simulink model "Sensor_fusion_4"  (R2024b)
settings: Solver=ode8  StartTime=0.0  StopTime=1000  FixedStep=0.1  RelTol=1e-3
values from neighbouring files (symbols this model uses):
  d = sqrt((Width/2)^2 + (Length/2)^2)    [VariableDeclare.m]
  Delta_t = 0.1    [VariableDeclare.m]
  Length = 0.5    [VariableDeclare.m]
  Wheel_radius = 0.1    [VariableDeclare.m]
  Width = 0.4    [VariableDeclare.m]
undefined symbols (not defined in the file or in its folder): DiscIntNeverNeededParam
libraries: ros2lib x3, simulink x3, sharedTrackingLibrary x1
settings Model: Creator=asrlab  LastModifiedBy=asrlab

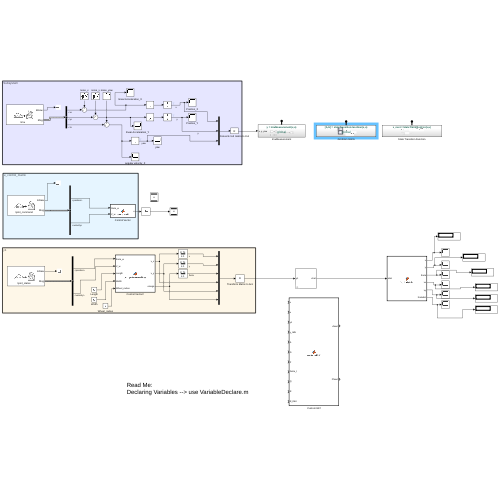
[thumbnail: Simulink's stored preview of the top-level diagram]
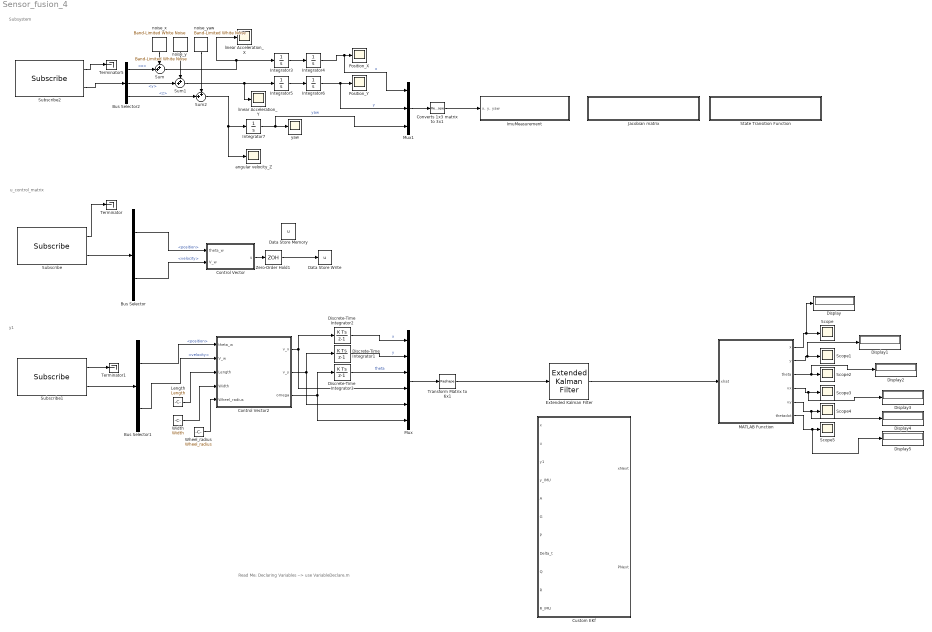
== system Sensor_fusion_4 ==
  note: Read Me:
      | Declaring Variables --> use VariableDeclare.m
  note: y1
  note: u_control_matrix
  note: Subsystem
  Bus Selector : BusSelector  OutputSignals=position,velocity
  Bus Selector1 : BusSelector  OutputSignals=position,velocity
  Bus Selector2 : BusSelector  OutputSignals=linear_acceleration.x,linear_acceleration.y,angular_velocity.z
  Control Vector : MATLAB Function  TreatAsAtomicUnit=on
  Control Vector2 : MATLAB Function  TreatAsAtomicUnit=on
  Converts 1x3 matrix to 3x1 : Reshape  OutputDimensionality=Customize  OutputDimensions=[3,1]
  Custom EKf : MATLAB Function  TreatAsAtomicUnit=on
  Data Store Memory : DataStoreMemory  DataStoreName=u  WriteAfterWriteMsg=warning  ShowAdditionalParam=off  OutDataTypeStr=double  Dimensions=[8 1]
  Data Store Write : DataStoreWrite  DataStoreName=u  IndexOptions=Index vector (dialog)  Indices=1  OutputSizes=1
  Discrete-Time Integrator1 : DiscreteIntegrator  SampleTime=-1  ICPrevOutput=DiscIntNeverNeededParam  ICPrevScaledInput=DiscIntNeverNeededParam
  Discrete-Time Integrator2 : DiscreteIntegrator  SampleTime=-1  ICPrevOutput=DiscIntNeverNeededParam  ICPrevScaledInput=DiscIntNeverNeededParam
  Discrete-Time Integrator3 : DiscreteIntegrator  SampleTime=-1  ICPrevOutput=DiscIntNeverNeededParam  ICPrevScaledInput=DiscIntNeverNeededParam
  Display{,1..5} (6 alike) : Display
  Extended Kalman Filter : sharedTrackingLibrary/Extended Kalman Filter  StateTransitionFcn=StateTransitionFcn  HasStateTransitionJacobianFcn=off  StateTransitionJacobianFcn=stateTransitionJacobian  HasAdditiveProcessNoise=Nonadditive  ProcessNoise=1  HasTimeVaryingProcessNoise=off  HasStateTransitionFcnExtraArgument=0  InitialState=initializationMatrix  InitialStateCovariance=P0  MeasurementFcn1=ImuMeasurement  HasMeasurementJacobianFcn1=off  HasMeasurementEnablePort1=off  HasAdditiveMeasurementNoise1=Nonadditive  MeasurementNoise1=R_IMU  HasTimeVaryingMeasurementNoise1=off  HasMeasurementFcnExtraArgument1=0  HasMeasurementWrapping1=off  MeasurementFcn2=myMeasurementFcn  HasMeasurementJacobianFcn2=off  HasMeasurementEnablePort2=off  HasAdditiveMeasurementNoise2=Additive  MeasurementNoise2=1  HasTimeVaryingMeasurementNoise2=off  HasMeasurementFcnExtraArgument2=0  HasMeasurementWrapping2=off  MeasurementFcn3=myMeasurementFcn  HasMeasurementJacobianFcn3=off  HasMeasurementEnablePort3=off  HasAdditiveMeasurementNoise3=Additive  MeasurementNoise3=1  HasTimeVaryingMeasurementNoise3=off  HasMeasurementFcnExtraArgument3=0  HasMeasurementWrapping3=off  MeasurementFcn4=myMeasurementFcn  HasMeasurementJacobianFcn4=off  HasMeasurementEnablePort4=off  HasAdditiveMeasurementNoise4=Additive  MeasurementNoise4=1  HasTimeVaryingMeasurementNoise4=off  HasMeasurementFcnExtraArgument4=0  HasMeasurementWrapping4=off  MeasurementFcn5=myMeasurementFcn  HasMeasurementJacobianFcn5=off  HasMeasurementEnablePort5=off  HasAdditiveMeasurementNoise5=Additive  MeasurementNoise5=1  HasTimeVaryingMeasurementNoise5=off  HasMeasurementFcnExtraArgument5=0  HasMeasurementWrapping5=off  EnableMultirate=off  StateTransitionFcnSampleTime=1  MeasurementFcn1SampleTime=1  MeasurementFcn2SampleTime=1  MeasurementFcn3SampleTime=1  MeasurementFcn4SampleTime=1  MeasurementFcn5SampleTime=1  UseCurrentEstimator=on  OutputStateCovariance=off  DataType=double  SampleTime=1  NumberOfMeasurements=1
  ImuMeasurement : Subsystem  TreatAsAtomicUnit=on
  Integrator{3..7} (5 alike) : Integrator
  Jacobian matrix : Subsystem  TreatAsAtomicUnit=on
  Length : Constant  Value=Length
  MATLAB Function : MATLAB Function  TreatAsAtomicUnit=on
  Mux : Mux  Inputs=6
  Mux1 : Mux  Inputs=3
  Position_X : Scope
  Position_Y : Scope
  Scope{,1..5} (6 alike) : Scope
  State Transition Function : Subsystem  TreatAsAtomicUnit=on
  Subscribe : ros2lib/Subscribe  topicSource=Select from ROS network  topic=/joint_command  messageType=sensor_msgs/JointState  sampleTime=-1  QOSHistory=Keep last  QOSDepth=1  QOSReliability=Reliable  QOSDurability=Volatile  QOSDeadline=Inf  QOSLifespan=Inf  QOSLiveliness=Automatic  QOSLeaseDuration=Inf  QOSAvoidROSNamespaceConventions=off
  Subscribe1 : ros2lib/Subscribe  topicSource=Select from ROS network  topic=/joint_states  messageType=sensor_msgs/JointState  sampleTime=-1  QOSHistory=Keep last  QOSDepth=1  QOSReliability=Reliable  QOSDurability=Volatile  QOSDeadline=Inf  QOSLifespan=Inf  QOSLiveliness=Automatic  QOSLeaseDuration=Inf  QOSAvoidROSNamespaceConventions=off
  Subscribe2 : ros2lib/Subscribe  topicSource=Select from ROS network  topic=/imu  messageType=sensor_msgs/Imu  sampleTime=-1  QOSHistory=Keep last  QOSDepth=1  QOSReliability=Reliable  QOSDurability=Volatile  QOSDeadline=Inf  QOSLifespan=Inf  QOSLiveliness=Automatic  QOSLeaseDuration=Inf  QOSAvoidROSNamespaceConventions=off
  Sum : Sum  Inputs=++|
  Sum1 : Sum  Inputs=++|
  Sum2 : Sum  Inputs=++|
  Terminator : Terminator
  Terminator1 : Terminator
  Terminator5 : Terminator
  Transform Matrix to 6x1 : Reshape  OutputDimensionality=Customize  OutputDimensions=[6,1]
  Wheel_radius : Constant  Value=Wheel_radius
  Width : Constant  Value=Width
  Zero-Order Hold1 : ZeroOrderHold  SampleTime=Delta_t
  angular velocity_Z : Scope
  linear Acceleration_X : Scope
  linear Acceleration_Y : Scope
  noise_x : simulink/Sources/Band-Limited White Noise  Cov=[0.1]  Ts=0.1  seed=[23341]
  noise_y : simulink/Sources/Band-Limited White Noise  Cov=[0.1]  Ts=0.1  seed=[23341]
  noise_yaw : simulink/Sources/Band-Limited White Noise  Cov=[0.1]  Ts=0.1  seed=[23341]
  yaw : Scope
  wires:
  Zero-Order Hold1/1 -> Data Store Write/1
  Control Vector/1(u) -> Zero-Order Hold1/1
  Bus Selector/1 -> Control Vector/1(theta_w)  "<position>"
  Subscribe/2 -> Bus Selector/1
  Bus Selector/2 -> Control Vector/2(V_w)  "<velocity>"
  Subscribe/1 -> Terminator/1
  Subscribe1/2 -> Bus Selector1/1
  Subscribe1/1 -> Terminator1/1
  Mux/1 -> Transform Matrix to 6x1/1
  Discrete-Time Integrator2/1 -> Mux/1  "x"
  Discrete-Time Integrator1/1 -> Mux/2  "y"
  Discrete-Time Integrator3/1 -> Mux/3  "theta"
  Integrator5/1 -> Integrator6/1
  Bus Selector2/3 -> Sum2/2  "<z>"
  Integrator4/1 -> Mux1/1, Position_X/1  "x"
  Sum2/1 -> Integrator7/1, angular velocity_Z/1
  Mux1/1 -> Converts 1x3 matrix to 3x1/1
  noise_yaw/1 -> Sum2/1
  Subscribe2/1 -> Terminator5/1
  noise_x/1 -> Sum/1
  Sum/1 -> Integrator3/1, linear Acceleration_X/1
  Integrator3/1 -> Integrator4/1
  Subscribe2/2 -> Bus Selector2/1
  noise_y/1 -> Sum1/1
  Bus Selector2/1 -> Sum/2  "<x>"
  Bus Selector2/2 -> Sum1/2  "<y>"
  Integrator7/1 -> Mux1/3, yaw/1  "yaw"
  Integrator6/1 -> Mux1/2, Position_Y/1  "y"
  Converts 1x3 matrix to 3x1/1 -> ImuMeasurement/1("x, y, yaw")
  Sum1/1 -> Integrator5/1, linear Acceleration_Y/1
  MATLAB Function/5(vy) -> Display4/1, Scope4/1
  MATLAB Function/4(vx) -> Display3/1, Scope3/1
  MATLAB Function/3(theta) -> Display2/1, Scope2/1
  MATLAB Function/2(y) -> Display1/1, Scope1/1
  MATLAB Function/6(thetadot) -> Display5/1, Scope5/1
  MATLAB Function/1(x) -> Display/1, Scope/1
  Width/1 -> Control Vector2/4(Width)
  Length/1 -> Control Vector2/3(Length)
  Bus Selector1/1 -> Control Vector2/1(theta_w)  "<position>"
  Bus Selector1/2 -> Control Vector2/2(V_w)  "<velocity>"
  Wheel_radius/1 -> Control Vector2/5(Wheel_radius)
  Control Vector2/1(v_x) -> Mux/4, Discrete-Time Integrator2/1
  Control Vector2/2(v_y) -> Mux/5, Discrete-Time Integrator1/1
  Control Vector2/3(omega) -> Mux/6, Discrete-Time Integrator3/1
  Transform Matrix to 6x1/1 -> Extended Kalman Filter/1
  Extended Kalman Filter/1 -> MATLAB Function/1(xhat)

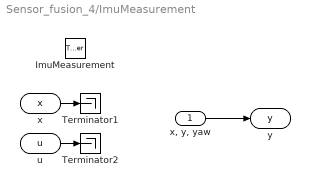
== system Sensor_fusion_4/ImuMeasurement ==
  "x, y, yaw" : Inport
  ImuMeasurement : TriggerPort  TriggerType=function-call  IsSimulinkFunction=on  FunctionName=ImuMeasurement  VariantControl=(inherit)
  Terminator1 : Terminator
  Terminator2 : Terminator
  x : ArgIn  DisableCoverage=on  PortDimensions=[6 1]  ArgumentName=x
  u : ArgIn  Port=2  PortDimensions=[8 1]  ArgumentName=u
  y : ArgOut  DisableCoverage=on  PortDimensions=3  ArgumentName=y
  wires:
  x/1 -> Terminator1/1
  u/1 -> Terminator2/1
  "x, y, yaw"/1 -> y/1

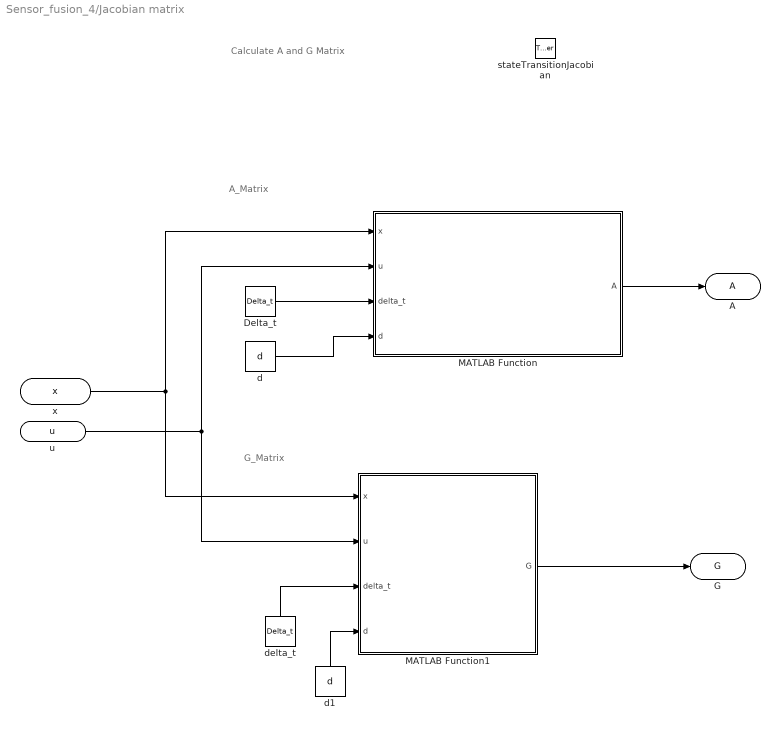
== system Sensor_fusion_4/Jacobian matrix ==
  note: Calculate A and G Matrix
  note: G_Matrix
  note: A_Matrix
  stateTransitionJacobian : TriggerPort  TriggerType=function-call  IsSimulinkFunction=on  FunctionName=stateTransitionJacobian  VariantControl=(inherit)
  Delta_t : Constant  Value=Delta_t
  MATLAB Function : MATLAB Function  TreatAsAtomicUnit=on
  MATLAB Function1 : MATLAB Function  TreatAsAtomicUnit=on
  d : Constant  Value=d
  d1 : Constant  Value=d
  delta_t : Constant  Value=Delta_t
  x : ArgIn  PortDimensions=[6 1]  ArgumentName=x
  u : ArgIn  Port=2  PortDimensions=[8 1]  ArgumentName=u
  A : ArgOut  DisableCoverage=on  PortDimensions=[6, 6]  ArgumentName=A
  G : ArgOut  DisableCoverage=on  Port=2  PortDimensions=[6, 8]  ArgumentName=G
  wires:
  MATLAB Function/1(A) -> A/1
  MATLAB Function1/1(G) -> G/1
  x/1 -> MATLAB Function1/1(x), MATLAB Function/1(x)
  u/1 -> MATLAB Function1/2(u), MATLAB Function/2(u)
  d/1 -> MATLAB Function/4(d)
  Delta_t/1 -> MATLAB Function/3(delta_t)
  d1/1 -> MATLAB Function1/4(d)
  delta_t/1 -> MATLAB Function1/3(delta_t)

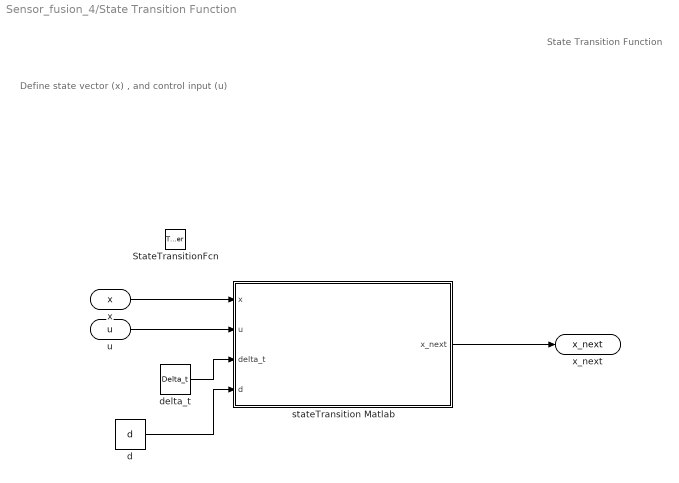
== system Sensor_fusion_4/State Transition Function ==
  note: Define state vector (x) , and control input (u)
  note: State Transition Function
  StateTransitionFcn : TriggerPort  TriggerType=function-call  IsSimulinkFunction=on  FunctionName=StateTransitionFcn  FunctionVisibility=scoped  VariantControl=(inherit)
  d : Constant  Value=d
  delta_t : Constant  Value=Delta_t
  stateTransition Matlab : MATLAB Function  TreatAsAtomicUnit=on
  x : ArgIn  DisableCoverage=on  PortDimensions=[6,1]  ArgumentName=x
  u : ArgIn  Port=2  ArgumentName=u
  x_next : ArgOut  DisableCoverage=on  PortDimensions=[6,1]  ArgumentName=x_next
  wires:
  stateTransition Matlab/1(x_next) -> x_next/1
  delta_t/1 -> stateTransition Matlab/3(delta_t)
  d/1 -> stateTransition Matlab/4(d)
  x/1 -> stateTransition Matlab/1(x)
  u/1 -> stateTransition Matlab/2(u)

== matlab function Sensor_fusion_4/Jacobian matrix/MATLAB Function ==
  data: x input; A output; u input; delta_t input; d input
function A = computeAMatrix(x, u, delta_t, d)
    % Extract state variables
    theta = x(3);      % Orientation
    v_x = x(4);        % Velocity in the x-direction
    v_y = x(5);        % Velocity in the y-direction
    omega = x(6);
    v = u(1:4);        % Velocities [v1, v2, v3, v4]
    delta = u(5:8);    % Steering angles [delta1, delta2, delta3, delta4]

    % Compute the summation term for the omega row
    sum_term = 0;
    for i = 1:4
        sum_term = sum_term + v(i) * cos(delta(i) - theta);
    end

    % Construct the A matrix
    A = [1, 0, (-v_x * sin(theta) - v_y * cos(theta)) * delta_t, cos(theta) * delta_t, -sin(theta) * delta_t, 0;
         0, 1, (v_x * cos(theta) - v_y * sin(theta)) * delta_t, sin(theta) * delta_t,  cos(theta) * delta_t, 0;
         0, 0, 1, 0, 0, delta_t;
         0, 0, 0, 1, 0, 0;
         0, 0, 0, 0, 1, 0;
         0, 0, omega, 0, 0, 1];
end

== matlab function Sensor_fusion_4/Control Vector2 ==
  data: theta_w input; v_x output; V_w input; v_y output; omega output; Length input; Width input; Wheel_radius input
function [v_x, v_y, omega] = computeVelocities(theta_w, V_w, Length, Width, Wheel_radius)
    % Compute the robot's linear velocities (v_x, v_y) and angular velocity (omega)
    % based on wheel velocities and steering angles from /joint_command.
    % - right_front_connector_joint
    % - left_front_connector_joint
    % - left_back_connector_joint
    % - right_back_connector_joint
    % - right_front_wheel_joint
    % - left_front_wheel_joint
    % - left_back_wheel_joint
    % - right_back_wheel_joint

    % theta_w: Vector of steering angles [theta1, theta2, theta3, theta4, thetawheel1,thetawheel2,thetawheel3, thetawheel4,]
    % V_w: Vector of wheel velocities [theta1, theta2, theta3, theta4, v1, v2, v3, v4]

    % Length: Distance between front and rear axles (wheelbase)
    % Width: Distance between left and right wheels (track width)
    % Length: Distance between front and rear axles (wheelbase)
    % Width: Distance between left and right wheels (track width)

    % Compute half dimensions for easier calculations
    L = Length / 2; % Half of the robot's length
    W = Width / 2;  % Half of the robot's width
    

    % Extract wheel speeds and angles
    speedRF = V_w(5);
    speedLF = V_w(6);
    speedLB = V_w(7);
    speedRB = V_w(8);
    angleRF = theta_w(1) + pi/2; % Adjust for -90 degrees (pi/2) skew
    angleLF = theta_w(2) + pi/2; % Adjust for -90 degrees (pi/2) skew
    angleLB = theta_w(3) + pi/2; % Adjust for -90 degrees (pi/2) skew
    angleRB = theta_w(4) + pi/2; % Adjust for -90 degrees (pi/2) skew


    % Compute velocity components for each wheel
    Vx_RF = speedRF * cos(angleRF);
    Vy_RF = speedRF * sin(angleRF);
    
    Vx_LF = speedLF * cos(angleLF);
    Vy_LF = speedLF * sin(angleLF);
    
    Vx_LB = speedLB * cos(angleLB);
    Vy_LB = speedLB * sin(angleLB);
    
    Vx_RB = speedRB * cos(angleRB);
    Vy_RB = speedRB * sin(angleRB);

    % Average translational velocities
    v_x = (Vx_RF + Vx_LF + Vx_LB + Vx_RB) / 4*Wheel_radius;
    v_y = (Vy_RF + Vy_LF + Vy_LB + Vy_RB) / 4*Wheel_radius;

    % Compute rotational velocity (omega)
    omega = ((-Vy_RF + Vy_LF + Vy_LB - Vy_RB) / (2 * L) + ...
             (Vx_RF + Vx_LF - Vx_LB - Vx_RB) / (2 * W)) / 4*Wheel_radius; 
end

== matlab function Sensor_fusion_4/State Transition Function/stateTransition Matlab ==
  data: x input; u input; x_next output; delta_t input; d input
function x_next = stateTransitionFcn(x, u, delta_t, d)
    
    % Extract control inputs
    v = u(1:4);   % v1, v2, v3, v4
    delta = u(5:8); % delta1, delta2, delta3, delta4
    x_k = x(1);
    y_k = x(2);
    theta_k = x(3);
    
    % Compute intermediate variables
    v_x = (1/4) * ((v(1) * cos(delta(1)) + v(2) * cos(delta(2)) + ...
               v(3) * cos(delta(3)) + v(4) * cos(delta(4))));

    v_y = (1/4) * ((v(1) * sin(delta(1)) + v(2) * sin(delta(2)) + ...
               v(3) * sin(delta(3)) + v(4) * sin(delta(4))));
    
    omega = (1 / (4 * d)) * (v(1) * sin(delta(1) - theta_k) + ...
                         v(2) * sin(delta(2) - theta_k) + ...
                         v(3) * sin(delta(3) - theta_k) + ...
                         v(4) * sin(delta(4) - theta_k));
    
    % Compute x_{k+1}, y_{k+1}, and theta_{k+1}
    x_next_x = x_k + v_x * delta_t * cos(theta_k) - v_y * delta_t * sin(theta_k);
    y_next_y = y_k + v_x * delta_t * sin(theta_k) + v_y * delta_t * cos(theta_k);
    theta_next = theta_k + omega * delta_t;
    
    % Compute velocity components
    v_x_next = v_x;
    v_y_next = v_y;
    omega_next = omega;
    
    % Combine into next state vector
    x_next = [x_next_x; y_next_y; theta_next; v_x_next; v_y_next; omega_next];
end

== matlab function Sensor_fusion_4/Jacobian matrix/MATLAB Function1 ==
  data: x input; G output; u input; delta_t input; d input
function G = computeGMatrix(x, u, delta_t, d)
    % Initialize the G matrix as a 6x8 matrix of zeros
    G = zeros(6, 8);

    % Extract control inputs from u
    v = u(1:4);        % Velocities [v1, v2, v3, v4]
    delta = u(5:8);    % Steering angles [delta1, delta2, delta3, delta4]

    % Extract state variables
    theta_k = x(3);    % Orientation

    % Compute each element of the G matrix using the given equations
    for i = 1:4
        % Partial derivatives with respect to v_i
        G(1, i) = (1/4) * (cos(delta(i)) * cos(theta_k) - sin(delta(i)) * sin(theta_k)) * delta_t; %Row 1 correct
        G(2, i) = (1/4) * (cos(delta(i)) * sin(theta_k) + sin(delta(i)) * cos(theta_k)) * delta_t; %Row 2 correct
        G(3, i) = (1 / (4 * d)) * sin(delta(i) - theta_k) * delta_t;
        G(4, i) = (1/4) * cos(delta(i));
        G(5, i) = (1/4) * sin(delta(i));
        G(6, i) = (1 / (4 * d)) * sin(delta(i) - theta_k);

        % Partial derivatives with respect to delta_i
        G(1, i + 4) = -(1/4) * v(i) * (sin(delta(i)) * cos(theta_k) + cos(delta(i)) * sin(theta_k)) * delta_t; 
        G(2, i + 4) = (1/4) * v(i) * (-sin(delta(i)) * sin(theta_k) + cos(delta(i)) * cos(theta_k)) * delta_t;
        G(3, i + 4) = (1 / (4 * d)) * v(i) * cos(delta(i) - theta_k) * delta_t;
        G(4, i + 4) = -(1/4) * v(i) * sin(delta(i));
        G(5, i + 4) = (1/4) * v(i) * cos(delta(i));
        G(6, i + 4) = (1 / (4 * d)) * v(i) * cos(delta(i) - theta_k);
    end
end

== matlab function Sensor_fusion_4/Control Vector ==
  data: theta_w input; u output; V_w input
function u = combineU(theta_w, V_w) % Subscribes from /joint_command to create the u matrix 
%!!!!!THE CONTROL VECTOR FOR /joint_states and/joint_commands are DIFFERENT!!!!!!

    % theta_w: Vector of steering angles [theta1, theta2, theta3, theta4 wheel_angle1 wheel_angle2 wheel_angle3 wheel_angle_4]T
    % V_w: Vector of wheel velocities [velocity_theta1 velocity_theta2 velocity_theta3 velocity_theta4 v1 v2 v3 v4]T
%#codegen    
    %Names: 
        % - right_front_connector_joint
        % - left_front_connector_joint
        % - left_back_connector_joint
        % - right_back_connector_joint
        % - right_front_wheel_joint
        % - left_front_wheel_joint
        % - left_back_wheel_joint
        % - right_back_wheel_joint
    % Define Control Vector u
    u = [   V_w(5);
            V_w(6); 
            V_w(7); 
            V_w(8);
            theta_w(1);
            theta_w(2);
            theta_w(3);
            theta_w(4);]
 
end

== matlab function Sensor_fusion_4/Custom EKf ==
  data: x input; u input; y1 input; y_IMU input; A input; G input; xNext output size=6; P input; Delta_t input; PNext output size=[6 6]; Q input; R input; R_IMU input
function [xNext, PNext] = customEKF(x, u, y1, y_IMU, A, G, P, Delta_t, Q, R, R_IMU)
    % Custom Extended Kalman Filter with additional IMU measurement update.

    %% Prediction Step
    % Predict the state
    x_pred =(A * x + G * u);
    
    % Predict the covariance
    P_pred = A * P * A' + Q;

    %% Primary Measurement Update
    % Define the measurement matrix H for the primary sensor (full 6 states)
    H = eye(6);  % Assuming y1 measures all 6 states directly
    y_pred = H * x_pred;                % Predicted measurement
    y_residual = y1 - y_pred;           % Innovation (residual)
    
    % Innovation covariance for primary sensor
    S1 = H * P_pred * H' + R;
    
    % Stabilize S1 if it is close to singular by adding a small value to the diagonal
    if rcond(S1) < 1e-12
        warning('S1 matrix is close to singular. Adjusting R for stability.');
        S1 = S1 + eye(6) * 1e-6;
    end
    
    % Kalman Gain for primary sensor
    K1 = P_pred * H' / S1;
    
    % Update state and covariance with primary sensor
    x_upd1 = x_pred + K1 * y_residual;
    P_upd1 = (eye(6) - K1 * H) * P_pred;

    %% IMU Measurement Update
    % Define the measurement matrix H_IMU for the IMU sensor (first 3 states only)
    H_IMU = [eye(3), zeros(3, 3)];  % IMU measures first 3 states
    y_IMU_pred = H_IMU * x_upd1;    % Predicted IMU measurement
    y_IMU_residual = y_IMU - y_IMU_pred;  % Innovation (residual) for IMU
    
    % Innovation covariance for IMU sensor
    S_IMU = H_IMU * P_upd1 * H_IMU' + R_IMU;
    
    % Stabilize S_IMU if it is close to singular by adding a small value to the diagonal
    if rcond(S_IMU) < 1e-12
        warning('S_IMU matrix is close to singular. Adjusting R_IMU for stability.');
        S_IMU = S_IMU + eye(3) * 1e-6;
    end
    
    % Kalman Gain for IMU sensor
    K_IMU = P_upd1 * H_IMU' / S_IMU;
    
    % Final state and covariance update with IMU
    xNext = x_upd1 + K_IMU * y_IMU_residual;
    PNext = (eye(6) - K_IMU * H_IMU) * P_upd1;

    %% Output Reshaping for Simulink Compatibility
    % Ensure output dimensions are explicit for Simulink
    xNext = reshape(xNext, [6, 1]);
    PNext = reshape(PNext, [6, 6]);
end

== matlab function Sensor_fusion_4/MATLAB Function ==
  data: x output; xhat input; y output; theta output; vx output; vy output; thetadot output
function [x, y, theta, vx, vy, thetadot] = SplitMatrix(xhat)
%#codegen
    x = xhat(1);
    y = xhat(2);
    theta= xhat(3);
    vx= xhat(4);
    vy= xhat(5);
    thetadot= xhat(6);
end
